simulink model "Ex1_virtualsub"  (R2021a)
settings: Solver=VariableStepAuto  StartTime=0.0  StopTime=10.0  RelTol=1e-3
settings Model: Creator=reemb  LastModifiedBy=reemb

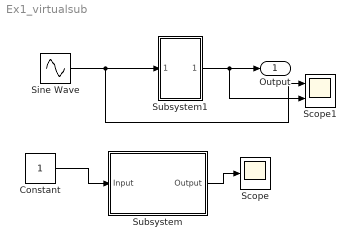
== system Ex1_virtualsub ==
  Constant : Constant
  Scope : Scope
  Scope1 : Scope  NumInputPorts=2
  Sine Wave : Sin  SampleTime=0
  Subsystem : Subsystem
  Subsystem1 : Subsystem
  Output : Outport
  wires:
  Constant/1 -> Subsystem/1(Input)
  Subsystem/1(Output) -> Scope/1
  Sine Wave/1 -> Scope1/1, Subsystem1/1(Input)
  Subsystem1/1(Output) -> Scope1/2, Output/1

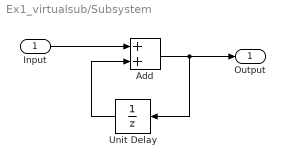
== system Ex1_virtualsub/Subsystem ==
  Input : Inport
  Add : Sum
  Unit Delay : UnitDelay  SampleTime=-1  HasFrameUpgradeWarning=on
  Output : Outport
  wires:
  Input/1 -> Add/1
  Unit Delay/1 -> Add/2
  Add/1 -> Output/1, Unit Delay/1

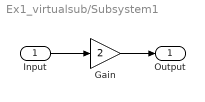
== system Ex1_virtualsub/Subsystem1 ==
  Input : Inport
  Gain : Gain  Gain=2
  Output : Outport
  wires:
  Gain/1 -> Output/1
  Input/1 -> Gain/1
